simulink model "vtol_pitch"  (R2020b)
settings: Solver=VariableStepAuto  StartTime=0.0  StopTime=30  RelTol=1e-3
values from neighbouring files (symbols this model uses):
  Ad = 1.175699206758237    (= 1.17569920676)    [VTOL_pitch_Simulink_constants.m]    (also in VTOL_roll_Simulink_constants.m = 1.1968251487; VTOL_yaw_Simulink_constants.m = 1.434674412)
  d = (rcp * dcp + rhp * dhp) / 2    (= 0.5715)    [VTOL_pitch_Simulink_constants.m]
  d_threshold = 1    [VTOL_pitch_Simulink_constants.m]    (also in VTOL_roll_Simulink_constants.m; VTOL_yaw_Simulink_constants.m)
  f = 0.517947467923121    (= 0.517947467923)    [VTOL_pitch_Simulink_constants.m]    (also in VTOL_roll_Simulink_constants.m = 0.625055192527; VTOL_yaw_Simulink_constants.m = 4.94171336132)
  Fmax = 71.22e3    (= 71220)    [VTOL_pitch_Simulink_constants.m]    (also in VTOL_roll_Simulink_constants.m)
  Jyy = Ixx + Izz    [VTOL_pitch_Simulink_constants.m]
  n_threshold = 1    [VTOL_pitch_Simulink_constants.m]    (also in VTOL_roll_Simulink_constants.m; VTOL_yaw_Simulink_constants.m)
  tau = 1/2    (= 0.5)    [VTOL_pitch_Simulink_constants.m]    (also in VTOL_roll_Simulink_constants.m)
libraries: simulink x1, pid_lib x1
settings Model: Creator=Tomo  LastModifiedBy=Tomo

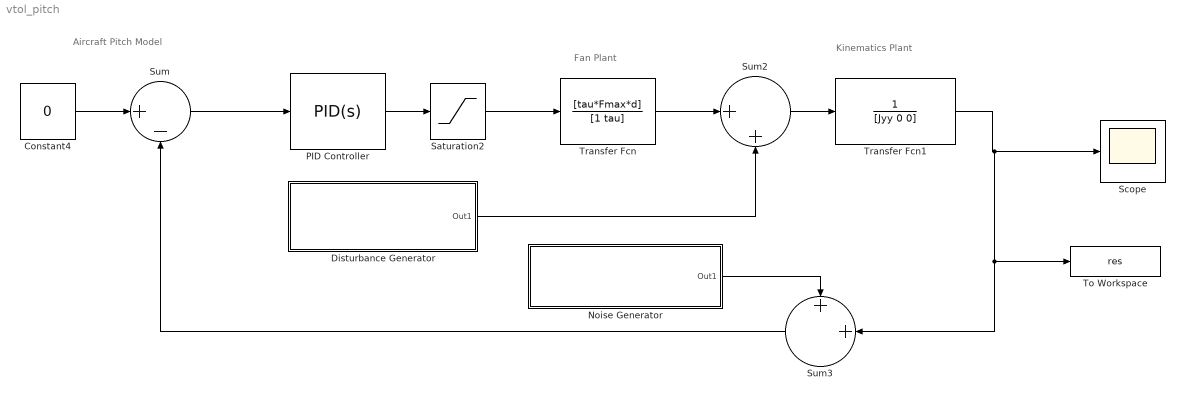
== system vtol_pitch ==
  note: Aircraft Pitch Model
  note: Kinematics Plant
  note: Fan Plant
  Constant4 : Constant  Value=0
  Disturbance Generator : Subsystem
  Noise Generator : Subsystem
  PID Controller : pid_lib/PID Controller  Controller=PID  Form=Parallel  TimeDomain=Continuous-time  UseExternalTs=off  SampleTime=-1  IntegratorMethod=Forward Euler  FilterMethod=Forward Euler  ControllerParametersSource=internal  P=2.11358067422841e-07  I=-9.70862952342768e-14  D=1.05676163147647  UseFilter=on  N=87.5084049402528  TunerSelectOption=Transfer Function Based (PID Tuner App)  InitialConditionSource=internal  InitialConditionForIntegrator=0  InitialConditionForFilter=0  DifferentiatorICPrevScaledInput=0  ExternalReset=none  TrackingMode=off  Kt=1  LimitOutput=off  SatLimitsSource=internal  UpperSaturationLimit=inf  LowerSaturationLimit=-inf  LinearizeAsGain=on  AntiWindupMode=none  Kb=1  POutMin=[]  POutMax=[]  IOutMin=[]  IOutMax=[]  DOutMin=[]  DOutMax=[]  NOutMin=[]  NOutMax=[]  SumOutMin=[]  SumOutMax=[]  SaturationOutMin=[]  SaturationOutMax=[]  PParamMin=[]  PParamMax=[]  IParamMin=[]  IParamMax=[]  DParamMin=[]  DParamMax=[]  NParamMin=[]  NParamMax=[]  KbParamMin=[]  KbParamMax=[]  KtParamMin=[]  KtParamMax=[]  KbOutMin=[]  KbOutMax=[]  KtOutMin=[]  KtOutMax=[]  IntegratorOutMin=[]  IntegratorOutMax=[]  FilterOutMin=[]  FilterOutMax=[]  SumI1OutMin=[]  SumI1OutMax=[]  SumI2OutMin=[]  SumI2OutMax=[]  SumI3OutMin=[]  SumI3OutMax=[]  SumI4OutMin=[]  SumI4OutMax=[]  SumDOutMin=[]  SumDOutMax=[]  DifferentiatorOutMin=[]  DifferentiatorOutMax=[]  FilterDiffOutCoefMin=[]  FilterDiffOutCoefMax=[]  ReciprocalOutMin=[]  ReciprocalOutMax=[]  SumDenOutMin=[]  SumDenOutMax=[]  SumNumOutMin=[]  SumNumOutMax=[]  DivideOutMin=[]  DivideOutMax=[]  UdiffTsProdOutMin=[]  UdiffTsProdOutMax=[]  NTsProdOutMin=[]  NTsProdOutMax=[]  UintegralTsProdOutMin=[]  UintegralTsProdOutMax=[]  UngainTsProdOutMin=[]  UngainTsProdOutMax=[]  IntegratorContinuousStateAttributes=''  IntegratorStateMustResolveToSignalObject=off  IntegratorRTWStateStorageClass=Auto  FilterContinuousStateAttributes=''  FilterStateMustResolveToSignalObject=off  FilterRTWStateStorageClass=Auto  ParallelPVariant=InternalParameters  IdealPVariant=Disabled  IVariant=InternalParameters  DVariant=InternalParameters  IntegratorVariant=Continuous  SatVariant=Disabled  AWVariant=Passthrough  PCopyVariant=Disabled  TRVariant=Disabled  FdbkBlocksVariant=Forward  IdealPFdbkVariant=Disabled  SatFdbkVariant=Disabled  DerivativeFilterVariant=ContFilter  NVariant=InternalParameters  NCopyVariant=Disabled  FilterICVariant=InternalICsFilter  IntegratorICVariant=InternalICs  ExternalResetVariant=Disabled  TRSumVariant=Passthrough  SumFdbkVariant=Disabled  SumVariant=Sum_PID  TsampFilterVariant=InternalTs  TsampNgainVariant=Passthrough  TsampIntegralVariant=Passthrough  ExternalSaturationOutDataTypeStr=Inherit: Same as second input
  Saturation2 : Saturate  UpperLimit=1  LowerLimit=-1  LinearizeAsGain=off
  Scope : Scope
  Sum : Sum  Inputs=|+-
  Sum2 : Sum  Inputs=|++
  Sum3 : Sum  Inputs=++|
  To Workspace : ToWorkspace  VariableName=res  SaveFormat=Structure With Time  SampleTime=-1
  Transfer Fcn : TransferFcn  Numerator=[tau*Fmax*d]  Denominator=[1 tau]
  Transfer Fcn1 : TransferFcn  Denominator=[Jyy 0 0]
  wires:
  Sum/1 -> PID Controller/1
  Transfer Fcn1/1 -> To Workspace/1, Sum3/2, Scope/1
  Sum2/1 -> Transfer Fcn1/1
  Sum3/1 -> Sum/2
  Transfer Fcn/1 -> Sum2/1
  PID Controller/1 -> Saturation2/1
  Saturation2/1 -> Transfer Fcn/1
  Disturbance Generator/1(Out1) -> Sum2/2
  Constant4/1 -> Sum/1
  Noise Generator/1(Out1) -> Sum3/1

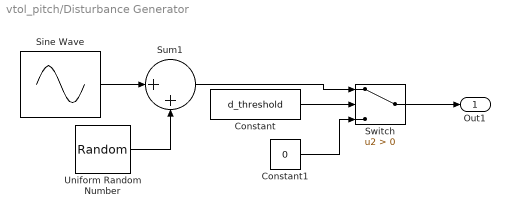
== system vtol_pitch/Disturbance Generator ==
  Constant : Constant  Value=d_threshold
  Constant1 : Constant  Value=0
  Sine Wave : Sin  Amplitude=Ad  Frequency=f*2*pi  SampleTime=0
  Sum1 : Sum  Inputs=|++
  Switch : Switch  Criteria=u2 > Threshold
  Uniform Random Number : UniformRandomNumber  SampleTime=0.1
  Out1 : Outport
  wires:
  Uniform Random Number/1 -> Sum1/2
  Sum1/1 -> Switch/1
  Sine Wave/1 -> Sum1/1
  Switch/1 -> Out1/1
  Constant/1 -> Switch/2
  Constant1/1 -> Switch/3

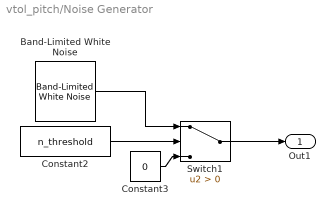
== system vtol_pitch/Noise Generator ==
  Band-Limited White Noise : simulink/Sources/Band-Limited White Noise  Cov=[0.1]  Ts=0.1  seed=[23341]
  Constant2 : Constant  Value=n_threshold
  Constant3 : Constant  Value=0
  Switch1 : Switch  Criteria=u2 > Threshold
  Out1 : Outport
  wires:
  Band-Limited White Noise/1 -> Switch1/1
  Constant2/1 -> Switch1/2
  Constant3/1 -> Switch1/3
  Switch1/1 -> Out1/1
